simulink model "VFA_ActModel1_2015a"  (R2015a)
settings: Solver=ode23tb  SolverMode=SingleTasking  StartTime=0.0  StopTime=tsim  FixedStep=0.001  RelTol=1e-3
values from neighbouring files (symbols this model uses):
  Aa_M = zeros([10,10,length(TP.etasweep)])    [SimVFA.m]
  Ba_aug_M = zeros([10,3,length(TP.etasweep)])    [SimVFA.m]
  Ba_M = zeros([10,2,length(TP.etasweep)])    [SimVFA.m]
  Bp = TP.B_hold(:,1:5,SO.eta_nom+1)    [SimVFA.m]
  Ca = [C, zeros(size(C,1),length(index_output)) ... (first row only)    [SimVFA.m]
  Caz_M = zeros([2,10,length(TP.etasweep)])    [SimVFA.m]
  Cz = [0,0,0,0,1,0,0,0 ... (first row only)    [SimVFA.m]
  K_M = zeros([2,10,length(TP.etasweep)])    [SimVFA.m]
  L_M = zeros([10,3,length(TP.etasweep)])    [SimVFA.m]
  Rinv_M = zeros([3,3,length(TP.etasweep)])    [SimVFA.m]
  S1_M = zeros([2,3,length(TP.etasweep)])    [SimVFA.m]
  S_M = zeros([3,3,length(TP.etasweep)])    [SimVFA.m]
undefined symbols (not defined in the file or in its folder): a10, a11, Aact, Acmd, Ada_Flag, ahold, Bact, Bact_x, Baz, Bcmd, Cact, Ccmd, d_sam, data, Gamma_l, Gamma_p1, Gamma_p2, Gamma_p21, i_input_sel, i_state_sel, initstate, input_hold, inputselect, lambda_0, Lambda_s, n_sam, psi1_0, psi21_0, psi2_0, samplet, Si1, Si2, state_hold, xm_0
libraries: simulink x8
settings Model: Creator=Travis  LastModifiedBy=ben
settings DataIOCC: SaveFormat=Structure  SignalLoggingSaveFormat=ModelDataLogs  SaveOutput=off  SignalLogging=off  DSMLogging=off  SaveTime=off  ReturnWorkspaceOutputs=on
settings OptimizationCC: BlockReduction=off  InlineParams=on  BufferReuse=off  ExpressionDepthLimit=2147483647  InitFltsAndDblsToZero=on
settings DebuggingCC: SaveWithParameterizedLinksMsg=none  UnderspecifiedInitializationDetection=Classic  MergeDetectMultiDrivingBlocksExec=none  SignalResolutionControl=TryResolveAllWithWarning  SolverPrmCheckMsg=warning  MultiTaskDSMMsg=warning  MultiTaskCondExecSysMsg=none  FcnCallInpInsideContextMsg=EnableAllAsWarning  StateNameClashWarn=warning  StrictBusMsg=Warning
settings GRTTargetCC: TargetFcnLib=ansi_tfl_tmw.mat  CombineOutputUpdateFcns=off  GRTInterface=on

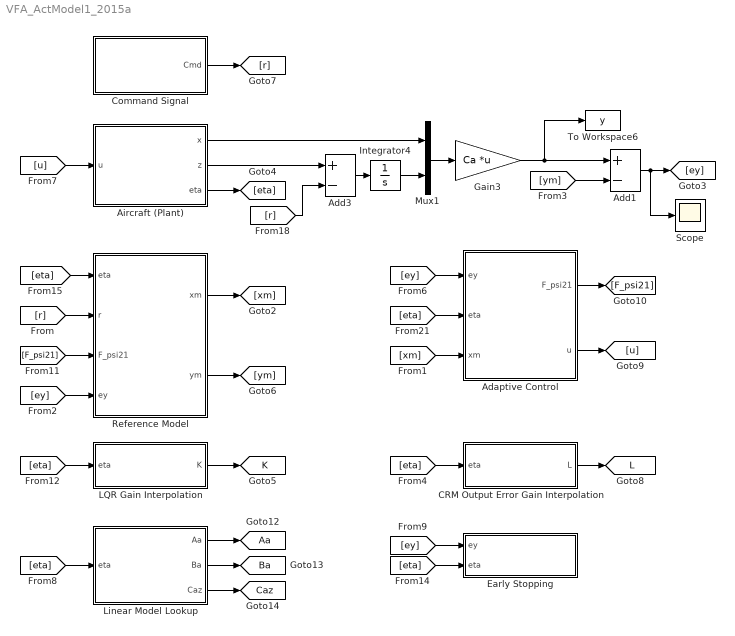
== system VFA_ActModel1_2015a ==
  Adaptive Control : Subsystem
  Add1 : Sum  Inputs=+-
  Add3 : Sum  Inputs=+-
  Aircraft (Plant) : Subsystem
  CRM Output Error Gain Interpolation : Subsystem
  Command Signal : Subsystem
  Early Stopping : Subsystem
  Gain3 : Gain  Gain=Ca  Multiplication=Matrix(K*u)
  Integrator4 : Integrator
  LQR Gain Interpolation : Subsystem
  Linear Model Lookup : Subsystem
  Mux1 : Mux  Inputs=2
  Reference Model : Subsystem
  Scope : Scope
      settings: TimeRange=auto  MaxDataPoints=5000  SaveToWorkspace=off  SaveName=ScopeData  YMin=-0.00038  YMax=0.00077  SampleTime=-1
  To Workspace6 : ToWorkspace  VariableName=y  SampleTime=-1
      settings: Decimation=data_deci
  tag scope: Aa=global, Ba=global, Caz=global, K=global, L=global
  wires:
  Command Signal/1(Cmd) -> [r]
  CRM Output Error Gain Interpolation/1(L) -> [L]
  Mux1/1 -> Gain3/1
  [ym] -> Add1/2
  Add1/1 -> Scope/1, [ey]
  [ey] -> Adaptive Control/1(ey)
  Adaptive Control/1(F_psi21) -> [F_psi21]
  Adaptive Control/2(u) -> [u]
  [eta] -> LQR Gain Interpolation/1(eta)
  [eta] -> Reference Model/1(eta)
  [r] -> Reference Model/2(r)
  [F_psi21] -> Reference Model/3(F_psi21)
  Reference Model/1(xm) -> [xm]
  Integrator4/1 -> Mux1/2
  [u] -> Aircraft (Plant)/1(u)
  Aircraft (Plant)/1(x) -> Mux1/1
  Add3/1 -> Integrator4/1
  Aircraft (Plant)/2(z) -> Add3/1
  [r] -> Add3/2
  LQR Gain Interpolation/1(K) -> [K]
  Reference Model/2(ym) -> [ym]
  Gain3/1 -> To Workspace6/1, Add1/1
  [xm] -> Adaptive Control/3(xm)
  Aircraft (Plant)/3(eta) -> [eta]
  [eta] -> CRM Output Error Gain Interpolation/1(eta)
  [eta] -> Adaptive Control/2(eta)
  [ey] -> Reference Model/4(ey)
  Linear Model Lookup/1(Aa) -> [Aa]
  Linear Model Lookup/2(Ba) -> [Ba]
  Linear Model Lookup/3(Caz) -> [Caz]
  [eta] -> Linear Model Lookup/1(eta)
  [eta] -> Early Stopping/2(eta)
  [ey] -> Early Stopping/1(ey)

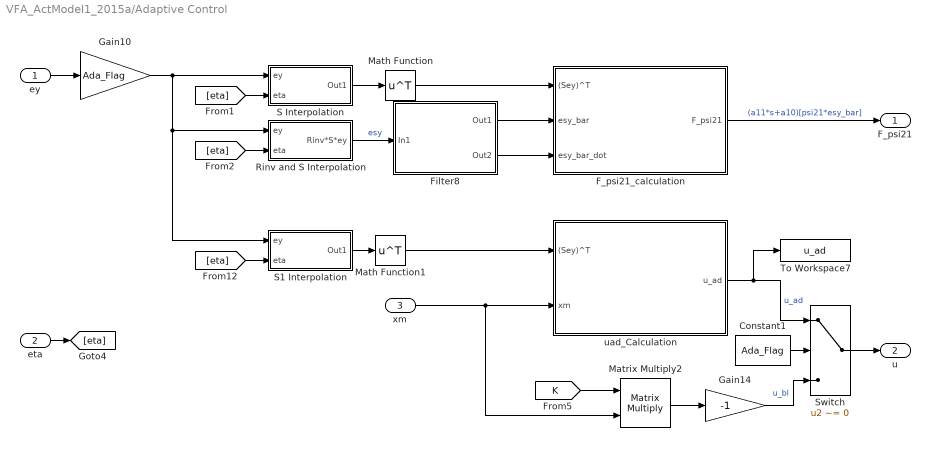
== system VFA_ActModel1_2015a/Adaptive Control ==
  ey : Inport
  eta : Inport  Port=2
  xm : Inport  Port=3
  Constant1 : Constant  Value=Ada_Flag  VectorParams1D=off
  F_psi21_calculation : Subsystem
  Filter8 : Subsystem
      mask Display: disp('NonUnit gain filters')
  Gain10 : Gain  Gain=Ada_Flag
  Gain14 : Gain  Gain=-1
  Math Function : Math  Operator=transpose  SaturateOnIntegerOverflow=on
  Math Function1 : Math  Operator=transpose  SaturateOnIntegerOverflow=on
  Matrix Multiply2 : Product  Multiplication=Matrix(*)
  Rinv and S Interpolation : Subsystem
  S Interpolation : Subsystem
  S1 Interpolation : Subsystem
  Switch : Switch  Criteria=u2 ~= 0
  To Workspace7 : ToWorkspace  VariableName=u_ad  SampleTime=-1
      settings: Decimation=data_deci
  uad_Calculation : Subsystem
  F_psi21 : Outport
  u : Outport  Port=2
  wires:
  S Interpolation/1(Out1) -> Math Function/1
  Math Function/1 -> F_psi21_calculation/1((Sey)^T)
  S1 Interpolation/1(Out1) -> Math Function1/1
  ey/1 -> Gain10/1
  uad_Calculation/1(u_ad) -> Switch/1, To Workspace7/1  "u_ad"
  F_psi21_calculation/1(F_psi21) -> F_psi21/1  "(a11*s+a10)[psi21*esy_bar]"
  xm/1 -> Matrix Multiply2/2, uad_Calculation/2(xm)
  eta/1 -> [eta]
  [eta] -> S1 Interpolation/2(eta)
  [eta] -> S Interpolation/2(eta)
  [eta] -> Rinv and S Interpolation/2(eta)
  Rinv and S Interpolation/1(Rinv*S*ey) -> Filter8/1(In1)  "esy"
  Filter8/1(Out1) -> F_psi21_calculation/2(esy_bar)
  Filter8/2(Out2) -> F_psi21_calculation/3(esy_bar_dot)
  Math Function1/1 -> uad_Calculation/1((Sey)^T)
  Constant1/1 -> Switch/2
  Switch/1 -> u/1
  Matrix Multiply2/1 -> Gain14/1
  Gain14/1 -> Switch/3  "u_bl"
  Gain10/1 -> S Interpolation/1(ey), S1 Interpolation/1(ey), Rinv and S Interpolation/1(ey)
  [K] -> Matrix Multiply2/1

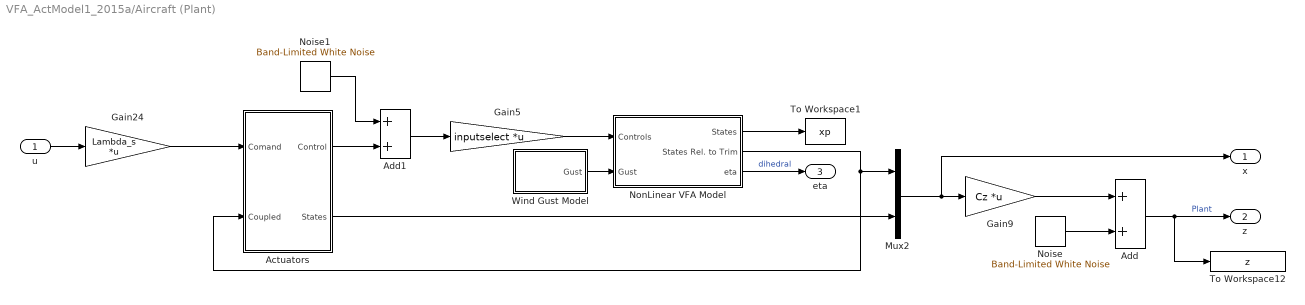
== system VFA_ActModel1_2015a/Aircraft (Plant) ==
  u : Inport
  Actuators : Subsystem
  Add : Sum
  Add1 : Sum  Inputs=2
  Gain24 : Gain  Gain=Lambda_s  Multiplication=Matrix(K*u)
  Gain5 : Gain  Gain=inputselect  Multiplication=Matrix(K*u)
  Gain9 : Gain  Gain=Cz  Multiplication=Matrix(K*u)
  Mux2 : Mux  Inputs=2
  Noise : simulink/Sources/Band-Limited White Noise  Cov=n_mean  Ts=n_sam  seed=n_seed
  Noise1 : simulink/Sources/Band-Limited White Noise  Cov=d_mean  Ts=d_sam  seed=d_seed
  NonLinear VFA Model : Subsystem
  To Workspace1 : ToWorkspace  VariableName=xp  SampleTime=-1
      settings: Decimation=data_deci
  To Workspace12 : ToWorkspace  VariableName=z  SampleTime=-1
      settings: Decimation=data_deci
  Wind Gust Model : Subsystem
  x : Outport
  z : Outport  Port=2
  eta : Outport  Port=3
  wires:
  Mux2/1 -> x/1, Gain9/1
  NonLinear VFA Model/2(States Rel. to Trim) -> Mux2/1, Actuators/2(Coupled)
  Gain9/1 -> Add/1
  Actuators/2(States) -> Mux2/2
  Add/1 -> To Workspace12/1, z/1  "Plant"
  Gain5/1 -> NonLinear VFA Model/1(Controls)
  NonLinear VFA Model/1(States) -> To Workspace1/1
  Wind Gust Model/1(Gust) -> NonLinear VFA Model/2(Gust)
  Gain24/1 -> Actuators/1(Comand)
  Noise/1 -> Add/2
  Noise1/1 -> Add1/1
  Actuators/1(Control) -> Add1/2
  Add1/1 -> Gain5/1
  u/1 -> Gain24/1
  NonLinear VFA Model/3(eta) -> eta/1  "dihedral"

== system VFA_ActModel1_2015a/CRM Output Error Gain Interpolation ==
  eta : Inport
  Constant2 : Constant  Value=L_M
  Gain : Gain  Gain=180/pi
  Subsystem1 : Subsystem
      mask Display: disp('matrix-interp');
  L : Outport
  wires:
  eta/1 -> Gain/1
  Subsystem1/1(Out1) -> L/1
  Gain/1 -> Subsystem1/1(In1)
  Constant2/1 -> Subsystem1/2(In2)

== system VFA_ActModel1_2015a/Command Signal ==
  Clock : Clock
  From Workspace : FromWorkspace  VariableName=r_timeseries  SampleTime=0  Interpolate=off  OutputAfterFinalValue=Holding final value
  To Workspace14 : ToWorkspace  VariableName=r_cmd  SampleTime=-1
      settings: Decimation=data_deci
  To Workspace6 : ToWorkspace  VariableName=t_sim  SampleTime=-1
      settings: Decimation=data_deci
  cmd filter : StateSpace  A=Acmd  B=Bcmd  C=Ccmd  D=zeros(size(Ccmd,1),size(Bcmd,2))  X0=0
  Cmd : Outport
  wires:
  Clock/1 -> To Workspace6/1
  cmd filter/1 -> To Workspace14/1, Cmd/1
  From Workspace/1 -> cmd filter/1

== system VFA_ActModel1_2015a/Early Stopping ==
  ey : Inport
  eta : Inport  Port=2
  Compare To Constant : simulink/Logic and Bit Operations/Compare To Constant  relop=>=  const=1e3  OutDataTypeStr=boolean
  Compare To Constant1 : simulink/Logic and Bit Operations/Compare To Constant  relop=>=  const=20  OutDataTypeStr=boolean
  Dot Product : DotProduct  InputSameDT=on  OutDataTypeStr=Inherit: Inherit via internal rule
  Gain : Gain  Gain=180/pi
  Logical Operator : Logic  Operator=OR  AllPortsSameDT=off  OutDataTypeStr=boolean
  Stop Simulation : Stop
  wires:
  Dot Product/1 -> Compare To Constant/1
  ey/1 -> Dot Product/2, Dot Product/1
  Logical Operator/1 -> Stop Simulation/1
  Compare To Constant/1 -> Logical Operator/1
  Compare To Constant1/1 -> Logical Operator/2
  eta/1 -> Gain/1
  Gain/1 -> Compare To Constant1/1

== system VFA_ActModel1_2015a/LQR Gain Interpolation ==
  eta : Inport
  Constant2 : Constant  Value=K_M
  Gain : Gain  Gain=180/pi
  Subsystem1 : Subsystem
      mask Display: disp('matrix-interp');
  K : Outport
  wires:
  eta/1 -> Gain/1
  Gain/1 -> Subsystem1/1(In1)
  Subsystem1/1(Out1) -> K/1
  Constant2/1 -> Subsystem1/2(In2)

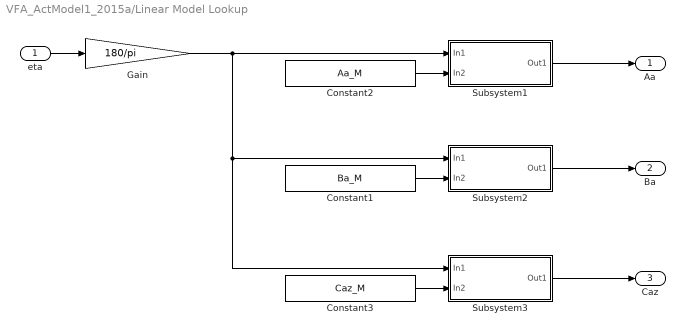
== system VFA_ActModel1_2015a/Linear Model Lookup ==
  eta : Inport
  Constant1 : Constant  Value=Ba_M
  Constant2 : Constant  Value=Aa_M
  Constant3 : Constant  Value=Caz_M
  Gain : Gain  Gain=180/pi
  Subsystem1 : Subsystem
      mask Display: disp('matrix-interp');
  Subsystem2 : Subsystem
      mask Display: disp('matrix-interp');
  Subsystem3 : Subsystem
      mask Display: disp('matrix-interp');
  Aa : Outport
  Ba : Outport  Port=2
  Caz : Outport  Port=3
  wires:
  eta/1 -> Gain/1
  Subsystem1/1(Out1) -> Aa/1
  Constant2/1 -> Subsystem1/2(In2)
  Constant1/1 -> Subsystem2/2(In2)
  Subsystem2/1(Out1) -> Ba/1
  Constant3/1 -> Subsystem3/2(In2)
  Gain/1 -> Subsystem1/1(In1), Subsystem3/1(In1), Subsystem2/1(In1)
  Subsystem3/1(Out1) -> Caz/1

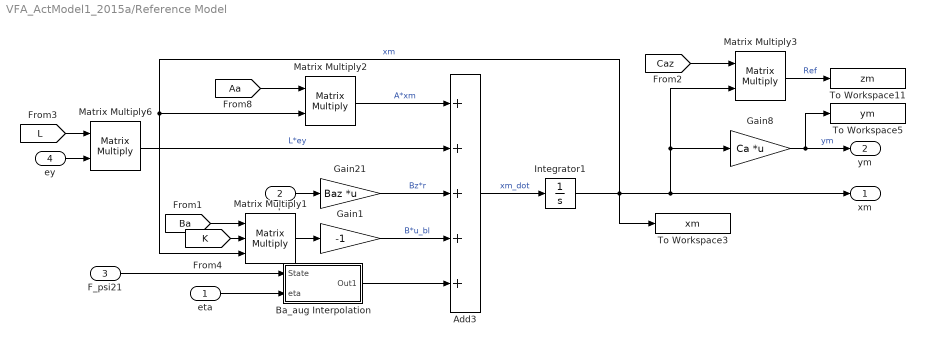
== system VFA_ActModel1_2015a/Reference Model ==
  eta : Inport
  r : Inport  Port=2
  F_psi21 : Inport  Port=3
  ey : Inport  Port=4
  Add3 : Sum  Inputs=+++++
  Ba_aug Interpolation : Subsystem
  Gain1 : Gain  Gain=-1
  Gain21 : Gain  Gain=Baz  Multiplication=Matrix(K*u)
  Gain8 : Gain  Gain=Ca  Multiplication=Matrix(K*u)
  Integrator1 : Integrator  InitialCondition=xm_0
  Matrix Multiply1 : Product  Inputs=3  Multiplication=Matrix(*)
  Matrix Multiply2 : Product  Multiplication=Matrix(*)
  Matrix Multiply3 : Product  Multiplication=Matrix(*)
  Matrix Multiply6 : Product  Multiplication=Matrix(*)
  To Workspace11 : ToWorkspace  VariableName=zm  SampleTime=-1
      settings: Decimation=data_deci
  To Workspace3 : ToWorkspace  VariableName=xm  SampleTime=-1
      settings: Decimation=data_deci
  To Workspace5 : ToWorkspace  VariableName=ym  SampleTime=-1
      settings: Decimation=data_deci
  xm : Outport
  ym : Outport  Port=2
  wires:
  Gain21/1 -> Add3/3  "Bz*r"
  Matrix Multiply2/1 -> Add3/1  "A*xm"
  Add3/1 -> Integrator1/1  "xm_dot"
  eta/1 -> Ba_aug Interpolation/2(eta)
  r/1 -> Gain21/1
  Gain1/1 -> Add3/4  "B*u_bl"
  Ba_aug Interpolation/1(Out1) -> Add3/5
  Matrix Multiply3/1 -> To Workspace11/1  "Ref"
  Gain8/1 -> ym/1, To Workspace5/1  "ym"
  Matrix Multiply6/1 -> Add3/2  "L*ey"
  ey/1 -> Matrix Multiply6/2
  F_psi21/1 -> Ba_aug Interpolation/1(State)
  [Aa] -> Matrix Multiply2/1
  Integrator1/1 -> To Workspace3/1, Matrix Multiply1/3, Matrix Multiply2/2, Matrix Multiply3/2, Gain8/1, xm/1  "xm"
  [Ba] -> Matrix Multiply1/1
  Matrix Multiply1/1 -> Gain1/1
  [K] -> Matrix Multiply1/2
  [Caz] -> Matrix Multiply3/1
  [L] -> Matrix Multiply6/1

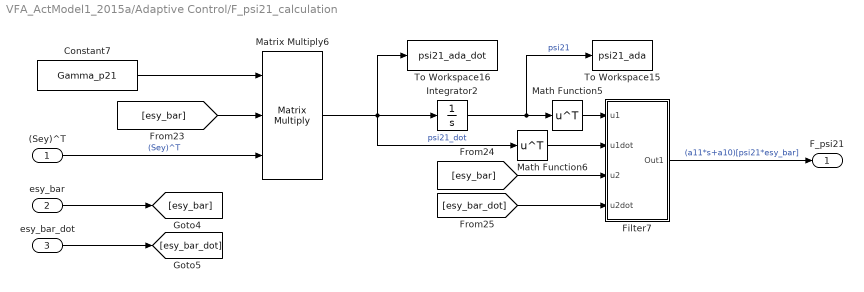
== system VFA_ActModel1_2015a/Adaptive Control/F_psi21_calculation ==
  (Sey)^T : Inport
  esy_bar : Inport  Port=2
  esy_bar_dot : Inport  Port=3
  Constant7 : Constant  Value=Gamma_p21  VectorParams1D=off
  Filter7 : Subsystem
      mask Display: disp('D1 Mixer')
  Integrator2 : Integrator  InitialCondition=psi21_0
  Math Function5 : Math  Operator=transpose  SaturateOnIntegerOverflow=on
  Math Function6 : Math  Operator=transpose  SaturateOnIntegerOverflow=on
  Matrix Multiply6 : Product  Inputs=3  Multiplication=Matrix(*)
  To Workspace15 : ToWorkspace  VariableName=psi21_ada  SampleTime=-1
      settings: Decimation=data_deci
  To Workspace16 : ToWorkspace  VariableName=psi21_ada_dot  SampleTime=-1
      settings: Decimation=data_deci
  F_psi21 : Outport
  wires:
  (Sey)^T/1 -> Matrix Multiply6/3  "(Sey)^T"
  Filter7/1(Out1) -> F_psi21/1  "(a11*s+a10)[psi21*esy_bar]"
  Integrator2/1 -> To Workspace15/1, Math Function5/1  "psi21"
  Math Function5/1 -> Filter7/1(u1)
  Constant7/1 -> Matrix Multiply6/1
  [esy_bar] -> Matrix Multiply6/2
  [esy_bar] -> Filter7/3(u2)
  Matrix Multiply6/1 -> To Workspace16/1, Math Function6/1, Integrator2/1  "psi21_dot"
  [esy_bar_dot] -> Filter7/4(u2dot)
  Math Function6/1 -> Filter7/2(u1dot)
  esy_bar_dot/1 -> [esy_bar_dot]
  esy_bar/1 -> [esy_bar]

== system VFA_ActModel1_2015a/Adaptive Control/Filter8 ==
  In1 : Inport
  Gain : Gain  Gain=a10/a11
  Gain1 : Gain
  Integrator : Integrator
  Sum : Sum  Inputs=|+-
  Out1 : Outport
  Out2 : Outport  Port=2
  wires:
  In1/1 -> Gain1/1
  Integrator/1 -> Out1/1, Gain/1
  Sum/1 -> Out2/1, Integrator/1
  Gain/1 -> Sum/2
  Gain1/1 -> Sum/1

== system VFA_ActModel1_2015a/Adaptive Control/Rinv and S Interpolation ==
  ey : Inport
  eta : Inport  Port=2
  Constant1 : Constant  Value=S_M
  Constant2 : Constant  Value=Rinv_M
  Gain : Gain  Gain=180/pi
  Gain1 : Gain  Gain=180/pi
  Matrix Multiply6 : Product  Inputs=3  Multiplication=Matrix(*)
  Subsystem1 : Subsystem
      mask Display: disp('matrix-interp');
  Subsystem2 : Subsystem
      mask Display: disp('matrix-interp');
  Rinv*S*ey : Outport
  wires:
  Subsystem1/1(Out1) -> Matrix Multiply6/1
  ey/1 -> Matrix Multiply6/3
  Matrix Multiply6/1 -> Rinv*S*ey/1
  Subsystem2/1(Out1) -> Matrix Multiply6/2
  Gain/1 -> Subsystem1/1(In1)
  Constant2/1 -> Subsystem1/2(In2)
  Gain1/1 -> Subsystem2/1(In1)
  Constant1/1 -> Subsystem2/2(In2)
  eta/1 -> Gain1/1, Gain/1

== system VFA_ActModel1_2015a/Adaptive Control/S Interpolation ==
  ey : Inport
  eta : Inport  Port=2
  Constant2 : Constant  Value=S_M
  Gain : Gain  Gain=180/pi
  Matrix Multiply6 : Product  Multiplication=Matrix(*)
  Subsystem1 : Subsystem
      mask Display: disp('matrix-interp');
  Out1 : Outport
  wires:
  eta/1 -> Gain/1
  Subsystem1/1(Out1) -> Matrix Multiply6/1
  ey/1 -> Matrix Multiply6/2
  Matrix Multiply6/1 -> Out1/1
  Gain/1 -> Subsystem1/1(In1)
  Constant2/1 -> Subsystem1/2(In2)

== system VFA_ActModel1_2015a/Adaptive Control/S1 Interpolation ==
  ey : Inport
  eta : Inport  Port=2
  Constant2 : Constant  Value=S1_M
  Gain : Gain  Gain=180/pi
  Matrix Multiply6 : Product  Multiplication=Matrix(*)
  Subsystem1 : Subsystem
      mask Display: disp('matrix-interp');
  Out1 : Outport
  wires:
  eta/1 -> Gain/1
  ey/1 -> Matrix Multiply6/2
  Matrix Multiply6/1 -> Out1/1
  Gain/1 -> Subsystem1/1(In1)
  Constant2/1 -> Subsystem1/2(In2)
  Subsystem1/1(Out1) -> Matrix Multiply6/1

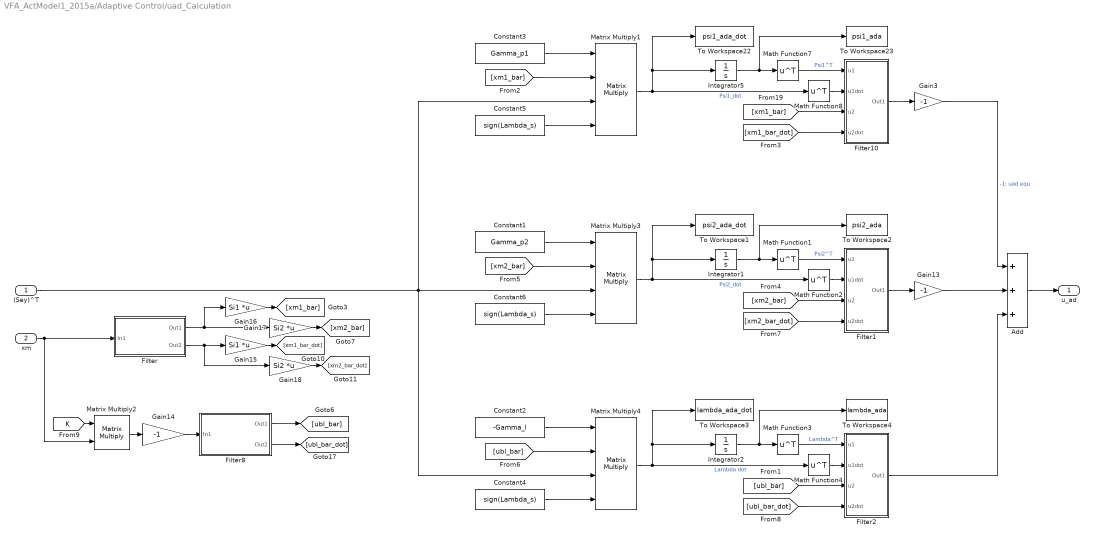
== system VFA_ActModel1_2015a/Adaptive Control/uad_Calculation ==
  (Sey)^T : Inport
  xm : Inport  Port=2
  Add : Sum  Inputs=3
  Constant1 : Constant  Value=Gamma_p2  VectorParams1D=off
  Constant2 : Constant  Value=-Gamma_l  VectorParams1D=off
  Constant3 : Constant  Value=Gamma_p1  VectorParams1D=off
  Constant4 : Constant  Value=sign(Lambda_s)  VectorParams1D=off
  Constant5 : Constant  Value=sign(Lambda_s)  VectorParams1D=off
  Constant6 : Constant  Value=sign(Lambda_s)  VectorParams1D=off
  Filter : Subsystem
      mask Display: disp('Unit gain filters')
  Filter1 : Subsystem
      mask Display: disp('D1 Mixer')
  Filter10 : Subsystem
      mask Display: disp('D1 Mixer')
  Filter2 : Subsystem
      mask Display: disp('D1 Mixer')
  Filter8 : Subsystem
      mask Display: disp('Unit gain filters')
  Gain13 : Gain  Gain=-1
  Gain14 : Gain  Gain=-1
  Gain15 : Gain  Gain=Si1  Multiplication=Matrix(K*u)
  Gain16 : Gain  Gain=Si1  Multiplication=Matrix(K*u)
  Gain17 : Gain  Gain=Si2  Multiplication=Matrix(K*u)
  Gain18 : Gain  Gain=Si2  Multiplication=Matrix(K*u)
  Gain3 : Gain  Gain=-1
  Integrator1 : Integrator  InitialCondition=psi2_0
  Integrator2 : Integrator  InitialCondition=lambda_0
  Integrator5 : Integrator  InitialCondition=psi1_0
  Math Function{1..4,7..8} (6 alike) : Math  Operator=transpose  SaturateOnIntegerOverflow=on
  Matrix Multiply1 : Product  Inputs=4  Multiplication=Matrix(*)
  Matrix Multiply2 : Product  Multiplication=Matrix(*)
  Matrix Multiply3 : Product  Inputs=4  Multiplication=Matrix(*)
  Matrix Multiply4 : Product  Inputs=4  Multiplication=Matrix(*)
  To Workspace1 : ToWorkspace  VariableName=psi2_ada_dot  SampleTime=-1
      settings: Decimation=data_deci
  To Workspace2 : ToWorkspace  VariableName=psi2_ada  SampleTime=-1
      settings: Decimation=data_deci
  To Workspace22 : ToWorkspace  VariableName=psi1_ada_dot  SampleTime=-1
      settings: Decimation=data_deci
  To Workspace23 : ToWorkspace  VariableName=psi1_ada  SampleTime=-1
      settings: Decimation=data_deci
  To Workspace3 : ToWorkspace  VariableName=lambda_ada_dot  SampleTime=-1
      settings: Decimation=data_deci
  To Workspace4 : ToWorkspace  VariableName=lambda_ada  SampleTime=-1
      settings: Decimation=data_deci
  u_ad : Outport
  wires:
  Gain13/1 -> Add/2
  Constant3/1 -> Matrix Multiply1/1
  [xm1_bar] -> Matrix Multiply1/2
  Filter10/1(Out1) -> Gain3/1
  Add/1 -> u_ad/1
  Gain3/1 -> Add/1  "-1: uad equ"
  Matrix Multiply2/1 -> Gain14/1
  [K] -> Matrix Multiply2/1
  Gain16/1 -> [xm1_bar]
  xm/1 -> Matrix Multiply2/2, Filter/1(In1)
  Filter8/1(Out1) -> [ubl_bar]
  Gain15/1 -> [xm1_bar_dot]
  Gain14/1 -> Filter8/1(In1)
  Filter/1(Out1) -> Gain17/1, Gain16/1
  Gain18/1 -> [xm2_bar_dot]
  Filter8/2(Out2) -> [ubl_bar_dot]
  Gain17/1 -> [xm2_bar]
  Filter/2(Out2) -> Gain15/1, Gain18/1
  Constant5/1 -> Matrix Multiply1/4
  [xm1_bar] -> Filter10/3(u2)
  Matrix Multiply1/1 -> Math Function8/1, Integrator5/1, To Workspace22/1  "Psi1_dot"
  Math Function8/1 -> Filter10/2(u1dot)
  Math Function7/1 -> Filter10/1(u1)  "Psi1^T"
  [xm1_bar_dot] -> Filter10/4(u2dot)
  Integrator5/1 -> To Workspace23/1, Math Function7/1
  [xm2_bar] -> Filter1/3(u2)
  Math Function2/1 -> Filter1/2(u1dot)
  Integrator1/1 -> To Workspace2/1, Math Function1/1
  Constant1/1 -> Matrix Multiply3/1
  Math Function1/1 -> Filter1/1(u1)  "Psi2^T"
  [xm2_bar_dot] -> Filter1/4(u2dot)
  Constant6/1 -> Matrix Multiply3/4
  [xm2_bar] -> Matrix Multiply3/2
  Matrix Multiply3/1 -> Math Function2/1, Integrator1/1, To Workspace1/1  "Psi2_dot"
  Filter1/1(Out1) -> Gain13/1
  Integrator2/1 -> To Workspace4/1, Math Function3/1
  [ubl_bar] -> Matrix Multiply4/2
  Constant4/1 -> Matrix Multiply4/4
  Math Function3/1 -> Filter2/1(u1)  "Lambda^T"
  Math Function4/1 -> Filter2/2(u1dot)
  [ubl_bar] -> Filter2/3(u2)
  Filter2/1(Out1) -> Add/3
  Constant2/1 -> Matrix Multiply4/1
  (Sey)^T/1 -> Matrix Multiply4/3, Matrix Multiply1/3, Matrix Multiply3/3
  Matrix Multiply4/1 -> Math Function4/1, Integrator2/1, To Workspace3/1  "Lambda dot"
  [ubl_bar_dot] -> Filter2/4(u2dot)

== system VFA_ActModel1_2015a/Aircraft (Plant)/Actuators ==
  Comand : Inport
  Coupled : Inport  Port=2
  Add : Sum  Inputs=3
  Gain1 : Gain  Gain=Bact  Multiplication=Matrix(K*u)
  Gain2 : Gain  Gain=Aact  Multiplication=Matrix(K*u)
  Gain3 : Gain  Gain=Bact_x  Multiplication=Matrix(K*u)
  Gain4 : Gain  Gain=Cact  Multiplication=Matrix(K*u)
  Integrator1 : Integrator
  Control : Outport
  States : Outport  Port=2
  wires:
  Gain1/1 -> Add/1
  Add/1 -> Integrator1/1
  Gain2/1 -> Add/2
  Integrator1/1 -> Gain4/1, Gain2/1
  Comand/1 -> Gain1/1
  Gain4/1 -> States/1, Control/1
  Coupled/1 -> Gain3/1
  Gain3/1 -> Add/3

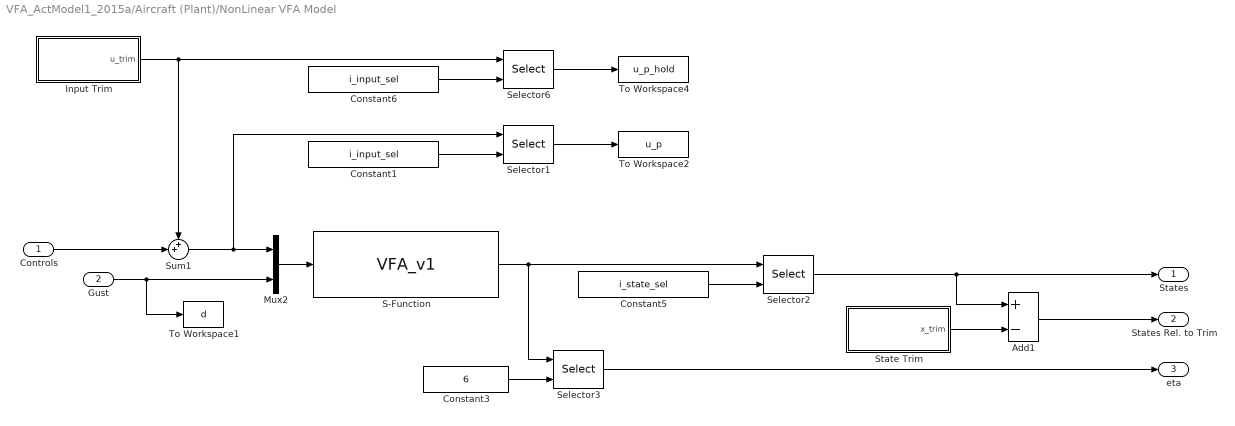
== system VFA_ActModel1_2015a/Aircraft (Plant)/NonLinear VFA Model ==
  Controls : Inport
  Gust : Inport  Port=2
  Add1 : Sum  Inputs=+-
  Constant1 : Constant  Value=i_input_sel
  Constant3 : Constant  Value=6
  Constant5 : Constant  Value=i_state_sel
  Constant6 : Constant  Value=i_input_sel
  Input Trim : Subsystem
  Mux2 : Mux  Inputs=2
  S-Function : S-Function  FunctionName=VFA_v1  Parameters=data,initstate  SFunctionDeploymentMode=off  EnableBusSupport=off
  Selector1 : Selector  InputPortWidth=size(Bp,2)  IndexOptions=Index vector (port)  Indices=[1 3]  OutputSizes=1
  Selector2 : Selector  InputPortWidth=length(Bp)  IndexOptions=Index vector (port)  Indices=[1 3]  OutputSizes=1
  Selector3 : Selector  InputPortWidth=length(Bp)  IndexOptions=Index vector (port)  Indices=[1 3]  OutputSizes=1
  Selector6 : Selector  InputPortWidth=size(Bp,2)  IndexOptions=Index vector (port)  Indices=[1 3]  OutputSizes=1
  State Trim : Subsystem
  Sum1 : Sum  Inputs=++|
  To Workspace1 : ToWorkspace  VariableName=d  SampleTime=-1
      settings: Decimation=data_deci
  To Workspace2 : ToWorkspace  VariableName=u_p  SampleTime=-1
      settings: Decimation=data_deci
  To Workspace4 : ToWorkspace  VariableName=u_p_hold  SampleTime=-1
      settings: Decimation=data_deci
  States : Outport
  States Rel. to Trim : Outport  Port=2
  eta : Outport  Port=3
  wires:
  Gust/1 -> To Workspace1/1, Mux2/2
  Mux2/1 -> S-Function/1
  Controls/1 -> Sum1/2
  Sum1/1 -> Selector1/1, Mux2/1
  Selector2/1 -> Add1/1, States/1
  Constant5/1 -> Selector2/2
  S-Function/1 -> Selector3/1, Selector2/1
  Constant1/1 -> Selector1/2
  Selector1/1 -> To Workspace2/1
  Constant3/1 -> Selector3/2
  Selector3/1 -> eta/1
  Input Trim/1(u_trim) -> Sum1/1, Selector6/1
  Constant6/1 -> Selector6/2
  Selector6/1 -> To Workspace4/1
  State Trim/1(x_trim) -> Add1/2
  Add1/1 -> States Rel. to Trim/1

== system VFA_ActModel1_2015a/Aircraft (Plant)/Wind Gust Model ==
  Band-Limited White Noise : simulink/Sources/Band-Limited White Noise  Cov=tpower  Ts=samplet  seed=[23341]
  Band-Limited White Noise1 : simulink/Sources/Band-Limited White Noise  Cov=tpower  Ts=samplet  seed=[23342]
  Band-Limited White Noise2 : simulink/Sources/Band-Limited White Noise  Cov=tpower  Ts=samplet  seed=[23345]
  Band-Limited White Noise3 : simulink/Sources/Band-Limited White Noise  Cov=tpower  Ts=samplet  seed=[23361]
  Mux5 : Mux
  Gust : Outport
  wires:
  Band-Limited White Noise/1 -> Mux5/1
  Band-Limited White Noise1/1 -> Mux5/2
  Band-Limited White Noise2/1 -> Mux5/3
  Band-Limited White Noise3/1 -> Mux5/4
  Mux5/1 -> Gust/1

== system VFA_ActModel1_2015a/CRM Output Error Gain Interpolation/Subsystem1 ==
  In1 : Inport
  In2 : Inport  Port=2
  Bias1 : Bias  Bias=1
  Direct Lookup Table (n-D)2 : LookupNDDirect  NumberOfTableDimensions=3  InputsSelectThisObjectFromTable=2-D Matrix  TableIsInput=on  Table=ahold
  Direct Lookup Table (n-D)3 : LookupNDDirect  NumberOfTableDimensions=3  InputsSelectThisObjectFromTable=2-D Matrix  TableIsInput=on  Table=ahold
  Fcn1 : Fcn  Expr=1-u(1)
  Prelookup1 : PreLookup  BreakpointsData=etasweep  ExtrapMethod=Linear
  Product2 : Product  RndMeth=Zero
  Product3 : Product  RndMeth=Zero
  Sum1 : Sum  Inputs=|++
  Out1 : Outport
  wires:
  In1/1 -> Prelookup1/1
  Sum1/1 -> Out1/1
  Prelookup1/1 -> Direct Lookup Table (n-D)3/1, Bias1/1
  Direct Lookup Table (n-D)2/1 -> Product2/1
  Prelookup1/2 -> Product2/2, Fcn1/1
  Direct Lookup Table (n-D)3/1 -> Product3/1
  Product2/1 -> Sum1/1
  Product3/1 -> Sum1/2
  Bias1/1 -> Direct Lookup Table (n-D)2/1
  In2/1 -> Direct Lookup Table (n-D)3/2, Direct Lookup Table (n-D)2/2
  Fcn1/1 -> Product3/2

== system VFA_ActModel1_2015a/LQR Gain Interpolation/Subsystem1 ==
  In1 : Inport
  In2 : Inport  Port=2
  Bias1 : Bias  Bias=1
  Direct Lookup Table (n-D)2 : LookupNDDirect  NumberOfTableDimensions=3  InputsSelectThisObjectFromTable=2-D Matrix  TableIsInput=on  Table=ahold
  Direct Lookup Table (n-D)3 : LookupNDDirect  NumberOfTableDimensions=3  InputsSelectThisObjectFromTable=2-D Matrix  TableIsInput=on  Table=ahold
  Fcn1 : Fcn  Expr=1-u(1)
  Prelookup1 : PreLookup  BreakpointsData=etasweep  ExtrapMethod=Linear
  Product2 : Product  RndMeth=Zero
  Product3 : Product  RndMeth=Zero
  Sum1 : Sum  Inputs=|++
  Out1 : Outport
  wires:
  In1/1 -> Prelookup1/1
  Sum1/1 -> Out1/1
  Prelookup1/1 -> Direct Lookup Table (n-D)3/1, Bias1/1
  Direct Lookup Table (n-D)2/1 -> Product2/1
  Prelookup1/2 -> Product2/2, Fcn1/1
  Direct Lookup Table (n-D)3/1 -> Product3/1
  Product2/1 -> Sum1/1
  Product3/1 -> Sum1/2
  Bias1/1 -> Direct Lookup Table (n-D)2/1
  In2/1 -> Direct Lookup Table (n-D)3/2, Direct Lookup Table (n-D)2/2
  Fcn1/1 -> Product3/2

== system VFA_ActModel1_2015a/Linear Model Lookup/Subsystem1 ==
  In1 : Inport
  In2 : Inport  Port=2
  Bias1 : Bias  Bias=1
  Direct Lookup Table (n-D)2 : LookupNDDirect  NumberOfTableDimensions=3  InputsSelectThisObjectFromTable=2-D Matrix  TableIsInput=on  Table=ahold
  Direct Lookup Table (n-D)3 : LookupNDDirect  NumberOfTableDimensions=3  InputsSelectThisObjectFromTable=2-D Matrix  TableIsInput=on  Table=ahold
  Fcn1 : Fcn  Expr=1-u(1)
  Prelookup1 : PreLookup  BreakpointsData=etasweep  ExtrapMethod=Linear
  Product2 : Product  RndMeth=Zero
  Product3 : Product  RndMeth=Zero
  Sum1 : Sum  Inputs=|++
  Out1 : Outport
  wires:
  In1/1 -> Prelookup1/1
  Sum1/1 -> Out1/1
  Prelookup1/1 -> Direct Lookup Table (n-D)3/1, Bias1/1
  Direct Lookup Table (n-D)2/1 -> Product2/1
  Prelookup1/2 -> Product2/2, Fcn1/1
  Direct Lookup Table (n-D)3/1 -> Product3/1
  Product2/1 -> Sum1/1
  Product3/1 -> Sum1/2
  Bias1/1 -> Direct Lookup Table (n-D)2/1
  In2/1 -> Direct Lookup Table (n-D)3/2, Direct Lookup Table (n-D)2/2
  Fcn1/1 -> Product3/2

== system VFA_ActModel1_2015a/Linear Model Lookup/Subsystem2 ==
  In1 : Inport
  In2 : Inport  Port=2
  Bias1 : Bias  Bias=1
  Direct Lookup Table (n-D)2 : LookupNDDirect  NumberOfTableDimensions=3  InputsSelectThisObjectFromTable=2-D Matrix  TableIsInput=on  Table=ahold
  Direct Lookup Table (n-D)3 : LookupNDDirect  NumberOfTableDimensions=3  InputsSelectThisObjectFromTable=2-D Matrix  TableIsInput=on  Table=ahold
  Fcn1 : Fcn  Expr=1-u(1)
  Prelookup1 : PreLookup  BreakpointsData=etasweep  ExtrapMethod=Linear
  Product2 : Product  RndMeth=Zero
  Product3 : Product  RndMeth=Zero
  Sum1 : Sum  Inputs=|++
  Out1 : Outport
  wires:
  In1/1 -> Prelookup1/1
  Sum1/1 -> Out1/1
  Prelookup1/1 -> Direct Lookup Table (n-D)3/1, Bias1/1
  Direct Lookup Table (n-D)2/1 -> Product2/1
  Prelookup1/2 -> Product2/2, Fcn1/1
  Direct Lookup Table (n-D)3/1 -> Product3/1
  Product2/1 -> Sum1/1
  Product3/1 -> Sum1/2
  Bias1/1 -> Direct Lookup Table (n-D)2/1
  In2/1 -> Direct Lookup Table (n-D)3/2, Direct Lookup Table (n-D)2/2
  Fcn1/1 -> Product3/2

== system VFA_ActModel1_2015a/Linear Model Lookup/Subsystem3 ==
  In1 : Inport
  In2 : Inport  Port=2
  Bias1 : Bias  Bias=1
  Direct Lookup Table (n-D)2 : LookupNDDirect  NumberOfTableDimensions=3  InputsSelectThisObjectFromTable=2-D Matrix  TableIsInput=on  Table=ahold
  Direct Lookup Table (n-D)3 : LookupNDDirect  NumberOfTableDimensions=3  InputsSelectThisObjectFromTable=2-D Matrix  TableIsInput=on  Table=ahold
  Fcn1 : Fcn  Expr=1-u(1)
  Prelookup1 : PreLookup  BreakpointsData=etasweep  ExtrapMethod=Linear
  Product2 : Product  RndMeth=Zero
  Product3 : Product  RndMeth=Zero
  Sum1 : Sum  Inputs=|++
  Out1 : Outport
  wires:
  In1/1 -> Prelookup1/1
  Sum1/1 -> Out1/1
  Prelookup1/1 -> Direct Lookup Table (n-D)3/1, Bias1/1
  Direct Lookup Table (n-D)2/1 -> Product2/1
  Prelookup1/2 -> Product2/2, Fcn1/1
  Direct Lookup Table (n-D)3/1 -> Product3/1
  Product2/1 -> Sum1/1
  Product3/1 -> Sum1/2
  Bias1/1 -> Direct Lookup Table (n-D)2/1
  In2/1 -> Direct Lookup Table (n-D)3/2, Direct Lookup Table (n-D)2/2
  Fcn1/1 -> Product3/2

== system VFA_ActModel1_2015a/Reference Model/Ba_aug Interpolation ==
  State : Inport
  eta : Inport  Port=2
  Constant2 : Constant  Value=Ba_aug_M
  Gain : Gain  Gain=180/pi
  Matrix Multiply6 : Product  Multiplication=Matrix(*)
  Subsystem1 : Subsystem
      mask Display: disp('matrix-interp');
  Out1 : Outport
  wires:
  eta/1 -> Gain/1
  Gain/1 -> Subsystem1/1(In1)
  Subsystem1/1(Out1) -> Matrix Multiply6/1
  State/1 -> Matrix Multiply6/2
  Matrix Multiply6/1 -> Out1/1
  Constant2/1 -> Subsystem1/2(In2)

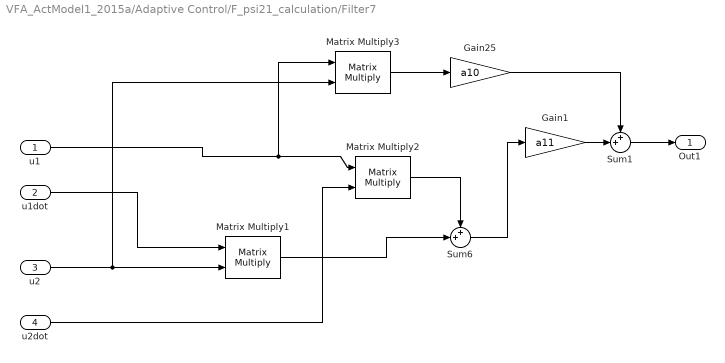
== system VFA_ActModel1_2015a/Adaptive Control/F_psi21_calculation/Filter7 ==
  u1 : Inport
  u1dot : Inport  Port=2
  u2 : Inport  Port=3
  u2dot : Inport  Port=4
  Gain1 : Gain  Gain=a11
  Gain25 : Gain  Gain=a10
  Matrix Multiply1 : Product  Multiplication=Matrix(*)
  Matrix Multiply2 : Product  Multiplication=Matrix(*)
  Matrix Multiply3 : Product  Multiplication=Matrix(*)
  Sum1 : Sum  Inputs=++|
  Sum6 : Sum  Inputs=++|
  Out1 : Outport
  wires:
  u1/1 -> Matrix Multiply3/1, Matrix Multiply2/1
  u2/1 -> Matrix Multiply3/2, Matrix Multiply1/2
  u1dot/1 -> Matrix Multiply1/1
  u2dot/1 -> Matrix Multiply2/2
  Matrix Multiply1/1 -> Sum6/2
  Matrix Multiply2/1 -> Sum6/1
  Sum6/1 -> Gain1/1
  Matrix Multiply3/1 -> Gain25/1
  Sum1/1 -> Out1/1
  Gain25/1 -> Sum1/1
  Gain1/1 -> Sum1/2

== system VFA_ActModel1_2015a/Adaptive Control/Rinv and S Interpolation/Subsystem1 ==
  In1 : Inport
  In2 : Inport  Port=2
  Bias1 : Bias  Bias=1
  Direct Lookup Table (n-D)2 : LookupNDDirect  NumberOfTableDimensions=3  InputsSelectThisObjectFromTable=2-D Matrix  TableIsInput=on  Table=ahold
  Direct Lookup Table (n-D)3 : LookupNDDirect  NumberOfTableDimensions=3  InputsSelectThisObjectFromTable=2-D Matrix  TableIsInput=on  Table=ahold
  Fcn1 : Fcn  Expr=1-u(1)
  Prelookup1 : PreLookup  BreakpointsData=etasweep  ExtrapMethod=Linear
  Product2 : Product  RndMeth=Zero
  Product3 : Product  RndMeth=Zero
  Sum1 : Sum  Inputs=|++
  Out1 : Outport
  wires:
  In1/1 -> Prelookup1/1
  Sum1/1 -> Out1/1
  Prelookup1/1 -> Direct Lookup Table (n-D)3/1, Bias1/1
  Direct Lookup Table (n-D)2/1 -> Product2/1
  Prelookup1/2 -> Product2/2, Fcn1/1
  Direct Lookup Table (n-D)3/1 -> Product3/1
  Product2/1 -> Sum1/1
  Product3/1 -> Sum1/2
  Bias1/1 -> Direct Lookup Table (n-D)2/1
  In2/1 -> Direct Lookup Table (n-D)3/2, Direct Lookup Table (n-D)2/2
  Fcn1/1 -> Product3/2

== system VFA_ActModel1_2015a/Adaptive Control/Rinv and S Interpolation/Subsystem2 ==
  In1 : Inport
  In2 : Inport  Port=2
  Bias1 : Bias  Bias=1
  Direct Lookup Table (n-D)2 : LookupNDDirect  NumberOfTableDimensions=3  InputsSelectThisObjectFromTable=2-D Matrix  TableIsInput=on  Table=ahold
  Direct Lookup Table (n-D)3 : LookupNDDirect  NumberOfTableDimensions=3  InputsSelectThisObjectFromTable=2-D Matrix  TableIsInput=on  Table=ahold
  Fcn1 : Fcn  Expr=1-u(1)
  Prelookup1 : PreLookup  BreakpointsData=etasweep  ExtrapMethod=Linear
  Product2 : Product  RndMeth=Zero
  Product3 : Product  RndMeth=Zero
  Sum1 : Sum  Inputs=|++
  Out1 : Outport
  wires:
  In1/1 -> Prelookup1/1
  Sum1/1 -> Out1/1
  Prelookup1/1 -> Direct Lookup Table (n-D)3/1, Bias1/1
  Direct Lookup Table (n-D)2/1 -> Product2/1
  Prelookup1/2 -> Product2/2, Fcn1/1
  Direct Lookup Table (n-D)3/1 -> Product3/1
  Product2/1 -> Sum1/1
  Product3/1 -> Sum1/2
  Bias1/1 -> Direct Lookup Table (n-D)2/1
  In2/1 -> Direct Lookup Table (n-D)3/2, Direct Lookup Table (n-D)2/2
  Fcn1/1 -> Product3/2

== system VFA_ActModel1_2015a/Adaptive Control/S Interpolation/Subsystem1 ==
  In1 : Inport
  In2 : Inport  Port=2
  Bias1 : Bias  Bias=1
  Direct Lookup Table (n-D)2 : LookupNDDirect  NumberOfTableDimensions=3  InputsSelectThisObjectFromTable=2-D Matrix  TableIsInput=on  Table=ahold
  Direct Lookup Table (n-D)3 : LookupNDDirect  NumberOfTableDimensions=3  InputsSelectThisObjectFromTable=2-D Matrix  TableIsInput=on  Table=ahold
  Fcn1 : Fcn  Expr=1-u(1)
  Prelookup1 : PreLookup  BreakpointsData=etasweep  ExtrapMethod=Linear
  Product2 : Product  RndMeth=Zero
  Product3 : Product  RndMeth=Zero
  Sum1 : Sum  Inputs=|++
  Out1 : Outport
  wires:
  In1/1 -> Prelookup1/1
  Sum1/1 -> Out1/1
  Prelookup1/1 -> Direct Lookup Table (n-D)3/1, Bias1/1
  Direct Lookup Table (n-D)2/1 -> Product2/1
  Prelookup1/2 -> Product2/2, Fcn1/1
  Direct Lookup Table (n-D)3/1 -> Product3/1
  Product2/1 -> Sum1/1
  Product3/1 -> Sum1/2
  Bias1/1 -> Direct Lookup Table (n-D)2/1
  In2/1 -> Direct Lookup Table (n-D)3/2, Direct Lookup Table (n-D)2/2
  Fcn1/1 -> Product3/2

== system VFA_ActModel1_2015a/Adaptive Control/S1 Interpolation/Subsystem1 ==
  In1 : Inport
  In2 : Inport  Port=2
  Bias1 : Bias  Bias=1
  Direct Lookup Table (n-D)2 : LookupNDDirect  NumberOfTableDimensions=3  InputsSelectThisObjectFromTable=2-D Matrix  TableIsInput=on  Table=ahold
  Direct Lookup Table (n-D)3 : LookupNDDirect  NumberOfTableDimensions=3  InputsSelectThisObjectFromTable=2-D Matrix  TableIsInput=on  Table=ahold
  Fcn1 : Fcn  Expr=1-u(1)
  Prelookup1 : PreLookup  BreakpointsData=etasweep  ExtrapMethod=Linear
  Product2 : Product  RndMeth=Zero
  Product3 : Product  RndMeth=Zero
  Sum1 : Sum  Inputs=|++
  Out1 : Outport
  wires:
  In1/1 -> Prelookup1/1
  Sum1/1 -> Out1/1
  Prelookup1/1 -> Direct Lookup Table (n-D)3/1, Bias1/1
  Direct Lookup Table (n-D)2/1 -> Product2/1
  Prelookup1/2 -> Product2/2, Fcn1/1
  Direct Lookup Table (n-D)3/1 -> Product3/1
  Product2/1 -> Sum1/1
  Product3/1 -> Sum1/2
  Bias1/1 -> Direct Lookup Table (n-D)2/1
  In2/1 -> Direct Lookup Table (n-D)3/2, Direct Lookup Table (n-D)2/2
  Fcn1/1 -> Product3/2

== system VFA_ActModel1_2015a/Adaptive Control/uad_Calculation/Filter ==
  In1 : Inport
  Gain : Gain  Gain=a10/a11
  Gain1 : Gain  Gain=a10/a11
  Integrator : Integrator
  Sum : Sum  Inputs=|+-
  Out1 : Outport
  Out2 : Outport  Port=2
  wires:
  In1/1 -> Gain/1
  Integrator/1 -> Out1/1, Gain1/1
  Sum/1 -> Out2/1, Integrator/1
  Gain/1 -> Sum/1
  Gain1/1 -> Sum/2

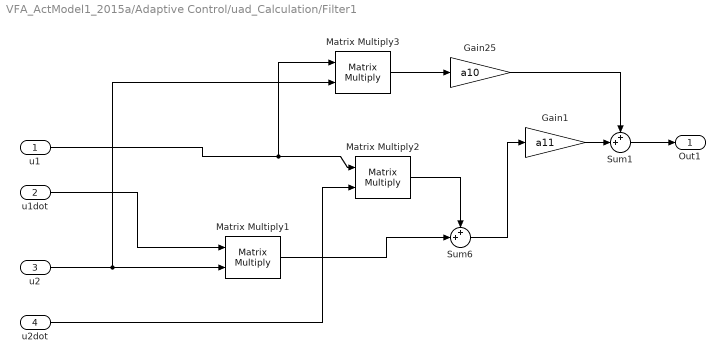
== system VFA_ActModel1_2015a/Adaptive Control/uad_Calculation/Filter1 ==
  u1 : Inport
  u1dot : Inport  Port=2
  u2 : Inport  Port=3
  u2dot : Inport  Port=4
  Gain1 : Gain  Gain=a11
  Gain25 : Gain  Gain=a10
  Matrix Multiply1 : Product  Multiplication=Matrix(*)
  Matrix Multiply2 : Product  Multiplication=Matrix(*)
  Matrix Multiply3 : Product  Multiplication=Matrix(*)
  Sum1 : Sum  Inputs=++|
  Sum6 : Sum  Inputs=++|
  Out1 : Outport
  wires:
  u1/1 -> Matrix Multiply3/1, Matrix Multiply2/1
  u2/1 -> Matrix Multiply3/2, Matrix Multiply1/2
  u1dot/1 -> Matrix Multiply1/1
  u2dot/1 -> Matrix Multiply2/2
  Matrix Multiply1/1 -> Sum6/2
  Matrix Multiply2/1 -> Sum6/1
  Sum6/1 -> Gain1/1
  Matrix Multiply3/1 -> Gain25/1
  Sum1/1 -> Out1/1
  Gain25/1 -> Sum1/1
  Gain1/1 -> Sum1/2

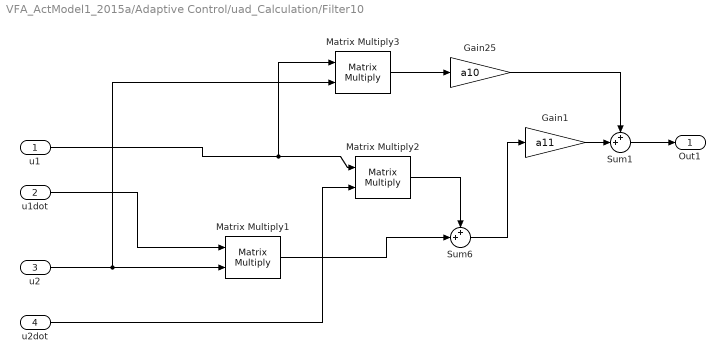
== system VFA_ActModel1_2015a/Adaptive Control/uad_Calculation/Filter10 ==
  u1 : Inport
  u1dot : Inport  Port=2
  u2 : Inport  Port=3
  u2dot : Inport  Port=4
  Gain1 : Gain  Gain=a11
  Gain25 : Gain  Gain=a10
  Matrix Multiply1 : Product  Multiplication=Matrix(*)
  Matrix Multiply2 : Product  Multiplication=Matrix(*)
  Matrix Multiply3 : Product  Multiplication=Matrix(*)
  Sum1 : Sum  Inputs=++|
  Sum6 : Sum  Inputs=++|
  Out1 : Outport
  wires:
  u1/1 -> Matrix Multiply3/1, Matrix Multiply2/1
  u2/1 -> Matrix Multiply3/2, Matrix Multiply1/2
  u1dot/1 -> Matrix Multiply1/1
  u2dot/1 -> Matrix Multiply2/2
  Matrix Multiply1/1 -> Sum6/2
  Matrix Multiply2/1 -> Sum6/1
  Sum6/1 -> Gain1/1
  Matrix Multiply3/1 -> Gain25/1
  Sum1/1 -> Out1/1
  Gain25/1 -> Sum1/1
  Gain1/1 -> Sum1/2

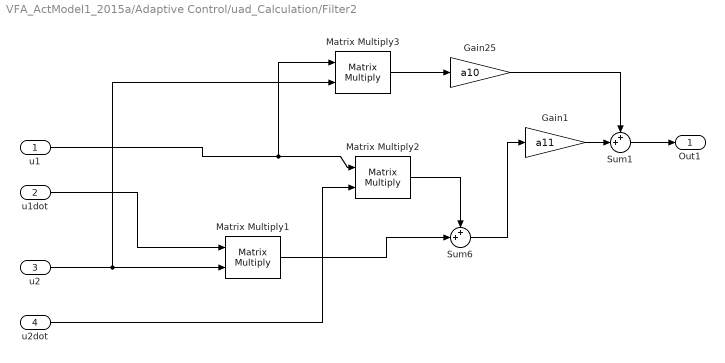
== system VFA_ActModel1_2015a/Adaptive Control/uad_Calculation/Filter2 ==
  u1 : Inport
  u1dot : Inport  Port=2
  u2 : Inport  Port=3
  u2dot : Inport  Port=4
  Gain1 : Gain  Gain=a11
  Gain25 : Gain  Gain=a10
  Matrix Multiply1 : Product  Multiplication=Matrix(*)
  Matrix Multiply2 : Product  Multiplication=Matrix(*)
  Matrix Multiply3 : Product  Multiplication=Matrix(*)
  Sum1 : Sum  Inputs=++|
  Sum6 : Sum  Inputs=++|
  Out1 : Outport
  wires:
  u1/1 -> Matrix Multiply3/1, Matrix Multiply2/1
  u2/1 -> Matrix Multiply3/2, Matrix Multiply1/2
  u1dot/1 -> Matrix Multiply1/1
  u2dot/1 -> Matrix Multiply2/2
  Matrix Multiply1/1 -> Sum6/2
  Matrix Multiply2/1 -> Sum6/1
  Sum6/1 -> Gain1/1
  Matrix Multiply3/1 -> Gain25/1
  Sum1/1 -> Out1/1
  Gain25/1 -> Sum1/1
  Gain1/1 -> Sum1/2

== system VFA_ActModel1_2015a/Adaptive Control/uad_Calculation/Filter8 ==
  In1 : Inport
  Gain1 : Gain  Gain=a10/a11
  Gain2 : Gain  Gain=a10/a11
  Integrator : Integrator
  Sum : Sum  Inputs=|+-
  Out1 : Outport
  Out2 : Outport  Port=2
  wires:
  In1/1 -> Gain1/1
  Integrator/1 -> Out1/1, Gain2/1
  Sum/1 -> Out2/1, Integrator/1
  Gain1/1 -> Sum/1
  Gain2/1 -> Sum/2

== system VFA_ActModel1_2015a/Aircraft (Plant)/NonLinear VFA Model/Input Trim ==
  Constant1 : Constant  Value=[1:5]
  Constant2 : Constant  Value=input_hold
  Selector1 : Selector  InputPortWidth=9  IndexOptions=Index vector (port)  Indices=[1 3]  OutputSizes=1
  u_trim : Outport
  wires:
  Constant1/1 -> Selector1/2
  Constant2/1 -> Selector1/1
  Selector1/1 -> u_trim/1

== system VFA_ActModel1_2015a/Aircraft (Plant)/NonLinear VFA Model/State Trim ==
  Constant3 : Constant  Value=state_hold
  Constant5 : Constant  Value=i_state_sel
  Selector2 : Selector  InputPortWidth=length(Bp)  IndexOptions=Index vector (port)  Indices=[1 3]  OutputSizes=1
  To Workspace3 : ToWorkspace  VariableName=x_hold  SampleTime=-1
      settings: Decimation=data_deci
  x_trim : Outport
  wires:
  Constant5/1 -> Selector2/2
  Constant3/1 -> Selector2/1
  Selector2/1 -> To Workspace3/1, x_trim/1

== system VFA_ActModel1_2015a/Reference Model/Ba_aug Interpolation/Subsystem1 ==
  In1 : Inport
  In2 : Inport  Port=2
  Bias1 : Bias  Bias=1
  Direct Lookup Table (n-D)2 : LookupNDDirect  NumberOfTableDimensions=3  InputsSelectThisObjectFromTable=2-D Matrix  TableIsInput=on  Table=ahold
  Direct Lookup Table (n-D)3 : LookupNDDirect  NumberOfTableDimensions=3  InputsSelectThisObjectFromTable=2-D Matrix  TableIsInput=on  Table=ahold
  Fcn1 : Fcn  Expr=1-u(1)
  Prelookup1 : PreLookup  BreakpointsData=etasweep  ExtrapMethod=Linear
  Product2 : Product  RndMeth=Zero
  Product3 : Product  RndMeth=Zero
  Sum1 : Sum  Inputs=|++
  Out1 : Outport
  wires:
  In1/1 -> Prelookup1/1
  Sum1/1 -> Out1/1
  Prelookup1/1 -> Direct Lookup Table (n-D)3/1, Bias1/1
  Direct Lookup Table (n-D)2/1 -> Product2/1
  Prelookup1/2 -> Product2/2, Fcn1/1
  Direct Lookup Table (n-D)3/1 -> Product3/1
  Product2/1 -> Sum1/1
  Product3/1 -> Sum1/2
  Bias1/1 -> Direct Lookup Table (n-D)2/1
  In2/1 -> Direct Lookup Table (n-D)3/2, Direct Lookup Table (n-D)2/2
  Fcn1/1 -> Product3/2
